simulink model "TCM16QAM_8AMPM"  (Simulink 10.2)
settings: Solver=VariableStepDiscrete  StartTime=0.0  StopTime=1000  RelTol=1e-3  EnableMultiTasking=on
model workspace (MAT data in the model file):
  A = 1
  BER_exit = 0.00293304002933
  BER_th = 0.001
  K = 8
  M = 16
  N = 51
  P_TCM = 10
  P_UNCODED = 10
  T = 1
  ber_TCM = [0.396503893847 0.381864367125 0.373007119222 0.359336876232 0.345566362512 0.327918713861 0.304321668505 0.274140178482 0.213543233397 0.100103613089 0.0215247835823 0.00237307396638 0.000300812192921 0]
  ber_UNCODED = [0.296470352965 0.274672532747 0.252474752525 0.224277572243 0.193513981935 0.163083691631 0.130453621305 0.101523181015 0.0726927307269 0.0482285104823 0.028797120288 0.0161650501617 0.00649935006499 0.00293304002933]
  ber_tcm_bit_coded = [0.462699288078 0.465055650256 0.463952672215 0.456833450316 0.452321267422 0.438884989472 0.415271232327 0.382382432568 0.324476085431 0.173568635315 0.0402085631204 0.00230622681239 0 0]
  ber_tcm_bit_uncoded = [0.2451011378 0.202749683944 0.169325153374 0.140053924506 0.107111756168 0.0906360906361 0.0594071533562 0.0492233646904 0.0336840162422 0.0120903805497 0.00424358158286 0.00165979277739 0.000451218289381 0]
  coded_bit = 3
  coded_bit_conv = [3 4]
  codegen = [1  0  0  0; 0  1  0  0; 0  0  133  171]
  codegen_2 = [133 171]
  constlen = [1 1 7]
  constlen_2 = 7
  generator_c1 = 133
  generator_c2 = 171
  h = 22
  hh = 0
  hws = Simulink.ModelWorkspace
  i = 15
  k = 3
  label_coded = 'TCM16QAM'
  label_uncoded = '8AMPM'
  list : struct (value not decoded)
  m = 4
  mapping_tcm = [-1-1i 3+3i -1+3i 3-1i -3-3i 1+1i -3+1i 1-3i -3+3i 1-1i -3-1i 1+3i -1+1i 3-3i -1-3i 3+1i]
  mapping_uncoded = [-1+3i -3+1i 3+3i 1+1i 3-1i 1-3i -1-1i -3-3i]
  mdl_name = 'TCM16QAM_8AMPM'
  mm = 0
  model = 'model_TCM16QAM_8AMPM'
  n = 10000
  num_states = 64
  register_length = 7
  seed = 208420
  snr = 14
  snr_start = 0
  snr_step = 1
  snr_vec = [0 1 2 3 4 5 6 7 8 9 10 11 12 13 14]
  ss = 0.824
  startTime = [2021 6 12 8 25 12.196]
  stepTime = [2021 6 12 8 25 35.192]
  step_dur = 0.824
  tb = 28
  tout = [9001 9002 9003 9004 9005 9006 9007 9008 9009 9010 9011 9012 ... (1000 elements, 1000x1)]
  trellis.numInputSymbols = 8
  trellis.numOutputSymbols = 16
  trellis.numStates = 64
  trellis.nextStates = [0  32  0  32  0  32  0  32; 0  32  0  32  0  32  0  32; 1  33  1  33  1  33  1  33; 1  33  1  33  1  33  1  33; 2  34  2  34  2  34  2  34; 2  34  2  34  2  34  2  34; 3  35  3  35  3  35  3  35; 3  35  3  35  3  35  3  35; 4  36  4  36  4  36  4  36; 4  36  4  36  4  36  4  36; 5  37  5  37  5  37  5  37; 5  37  5  37  5  37  5  37; 6  38  6  38  6  38  6  38; 6  38  6  38  6  38  6  38; 7  39  7  39  7  39  7  39; 7  39  7  39  7  39  7  39; 8  40  8  40  8  40  8  40; 8  40  8  40  8  40  8  40; 9  41  9  41  9  41  9  41; 9  41  9  41  9  41  9  41; 10  42  10  42  10  42  10  42; 10  42  10  42  10  42  10  42; 11  43  11  43  11  43  11  43; 11  43  11  43  11  43  11  43; 12  44  12  44  12  44  12  44; 12  44  12  44  12  44  12  44; 13  45  13  45  13  45  13  45; 13  45  13  45  13  45  13  45; 14  46  14  46  14  46  14  46; 14  46  14  46  14  46  14  46; 15  47  15  47  15  47  15  47; 15  47  15  47  15  47  15  47; 16  48  16  48  16  48  16  48; 16  48  16  48  16  48  16  48; 17  49  17  49  17  49  17  49; 17  49  17  49  17  49  17  49; 18  50  18  50  18  50  18  50; 18  50  18  50  18  50  18  50; 19  51  19  51  19  51  19  51; 19  51  19  51  19  51  19  51; 20  52  20  52  20  52  20  52; 20  52  20  52  20  52  20  52; 21  53  21  53  21  53  21  53; 21  53  21  53  21  53  21  53; 22  54  22  54  22  54  22  54; 22  54  22  54  22  54  22  54; 23  55  23  55  23  55  23  55; 23  55  23  55  23  55  23  55; 24  56  24  56  24  56  24  56; 24  56  24  56  24  56  24  56; 25  57  25  57  25  57  25  57; 25  57  25  57  25  57  25  57; 26  58  26  58  26  58  26  58; 26  58  26  58  26  58  26  58; 27  59  27  59  27  59  27  59; 27  59  27  59  27  59  27  59; 28  60  28  60  28  60  28  60; 28  60  28  60  28  60  28  60; 29  61  29  61  29  61  29  61; 29  61  29  61  29  61  29  61; 30  62  30  62  30  62  30  62; 30  62  30  62  30  62  30  62; 31  63  31  63  31  63  31  63; 31  63  31  63  31  63  31  63]
  trellis.outputs = [0  3  4  7  10  13  14  17; 3  0  7  4  13  10  17  14; 2  1  6  5  12  11  16  15; 1  2  5  6  11  12  15  16; 0  3  4  7  10  13  14  17; 3  0  7  4  13  10  17  14; 2  1  6  5  12  11  16  15; 1  2  5  6  11  12  15  16; 3  0  7  4  13  10  17  14; 0  3  4  7  10  13  14  17; 1  2  5  6  11  12  15  16; 2  1  6  5  12  11  16  15; 3  0  7  4  13  10  17  14; 0  3  4  7  10  13  14  17; 1  2  5  6  11  12  15  16; 2  1  6  5  12  11  16  15; 3  0  7  4  13  10  17  14; 0  3  4  7  10  13  14  17; 1  2  5  6  11  12  15  16; 2  1  6  5  12  11  16  15; 3  0  7  4  13  10  17  14; 0  3  4  7  10  13  14  17; 1  2  5  6  11  12  15  16; 2  1  6  5  12  11  16  15; 0  3  4  7  10  13  14  17; 3  0  7  4  13  10  17  14; 2  1  6  5  12  11  16  15; 1  2  5  6  11  12  15  16; 0  3  4  7  10  13  14  17; 3  0  7  4  13  10  17  14; 2  1  6  5  12  11  16  15; 1  2  5  6  11  12  15  16; 1  2  5  6  11  12  15  16; 2  1  6  5  12  11  16  15; 3  0  7  4  13  10  17  14; 0  3  4  7  10  13  14  17; 1  2  5  6  11  12  15  16; 2  1  6  5  12  11  16  15; 3  0  7  4  13  10  17  14; 0  3  4  7  10  13  14  17; 2  1  6  5  12  11  16  15; 1  2  5  6  11  12  15  16; 0  3  4  7  10  13  14  17; 3  0  7  4  13  10  17  14; 2  1  6  5  12  11  16  15; 1  2  5  6  11  12  15  16; 0  3  4  7  10  13  14  17; 3  0  7  4  13  10  17  14; 2  1  6  5  12  11  16  15; 1  2  5  6  11  12  15  16; 0  3  4  7  10  13  14  17; 3  0  7  4  13  10  17  14; 2  1  6  5  12  11  16  15; 1  2  5  6  11  12  15  16; 0  3  4  7  10  13  14  17; 3  0  7  4  13  10  17  14; 1  2  5  6  11  12  15  16; 2  1  6  5  12  11  16  15; 3  0  7  4  13  10  17  14; 0  3  4  7  10  13  14  17; 1  2  5  6  11  12  15  16; 2  1  6  5  12  11  16  15; 3  0  7  4  13  10  17  14; 0  3  4  7  10  13  14  17]
  trellis_2.numInputSymbols = 2
  trellis_2.numOutputSymbols = 4
  trellis_2.numStates = 64
  trellis_2.nextStates = [0  32; 0  32; 1  33; 1  33; 2  34; 2  34; 3  35; 3  35; 4  36; 4  36; 5  37; 5  37; 6  38; 6  38; 7  39; 7  39; 8  40; 8  40; 9  41; 9  41; 10  42; 10  42; 11  43; 11  43; 12  44; 12  44; 13  45; 13  45; 14  46; 14  46; 15  47; 15  47; 16  48; 16  48; 17  49; 17  49; 18  50; 18  50; 19  51; 19  51; 20  52; 20  52; 21  53; 21  53; 22  54; 22  54; 23  55; 23  55; 24  56; 24  56; 25  57; 25  57; 26  58; 26  58; 27  59; 27  59; 28  60; 28  60; 29  61; 29  61; 30  62; 30  62; 31  63; 31  63]
  trellis_2.outputs = [0  3; 3  0; 2  1; 1  2; 0  3; 3  0; 2  1; 1  2; 3  0; 0  3; 1  2; 2  1; 3  0; 0  3; 1  2; 2  1; 3  0; 0  3; 1  2; 2  1; 3  0; 0  3; 1  2; 2  1; 0  3; 3  0; 2  1; 1  2; 0  3; 3  0; 2  1; 1  2; 1  2; 2  1; 3  0; 0  3; 1  2; 2  1; 3  0; 0  3; 2  1; 1  2; 0  3; 3  0; 2  1; 1  2; 0  3; 3  0; 2  1; 1  2; 0  3; 3  0; 2  1; 1  2; 0  3; 3  0; 1  2; 2  1; 3  0; 0  3; 1  2; 2  1; 3  0; 0  3]
  uncoded_bit = [1 2]
undefined symbols (not defined in the file): Mnum
libraries: commsink2 x4, commutil2 x4, dspindex x4, commdigbbndam3 x3, commchan3 x2, commcnvcod2 x2, commdigbbndtcm2 x1, commrandsrc2 x1
settings Model: Creator=Diego  LastModifiedBy=diego
settings DataIOCC: LimitDataPoints=on
settings OptimizationCC: ExpressionDepthLimit=2147483647
settings DebuggingCC: SolverPrmCheckMsg=warning  StateNameClashWarn=warning
settings GRTTargetCC: CombineOutputUpdateFcns=on  GRTInterface=off

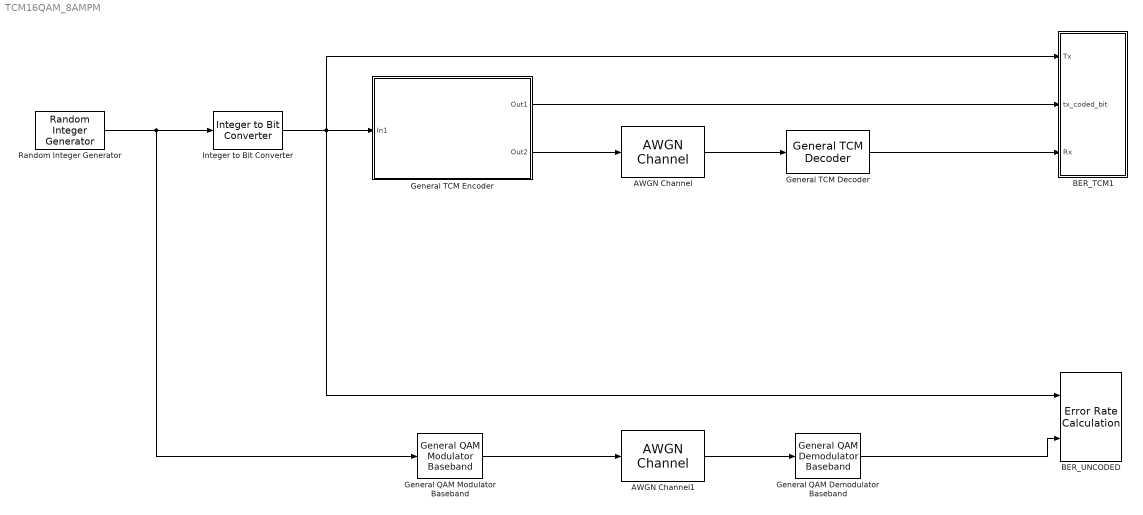
== system TCM16QAM_8AMPM ==
  AWGN Channel : commchan3/AWGN Channel  InputProcessing=Columns as channels (frame based)  seed=seed  noiseMode="Signal to noise ratio  (Es/No)"  EbNodB=Eb_No  EsNodB=snr  SNRdB=snr  bitsPerSym=k  Ps=P_TCM  Tsym=T  variance=1
  AWGN Channel1 : commchan3/AWGN Channel  InputProcessing=Columns as channels (frame based)  seed=seed  noiseMode="Signal to noise ratio  (Es/No)"  EbNodB=Eb_No  EsNodB=snr  SNRdB=snr  bitsPerSym=k  Ps=P_UNCODED  Tsym=1  variance=1
  BER_TCM1 : Subsystem
  BER_UNCODED : commsink2/Error Rate Calculation  N=0  st_delay=0  cp_mode=Entire frame  subframe=[]  PMode=Workspace  WsName=ErrorVec_UNCODED  RsMode2=off  stop=off  numErr=100  maxBits=1e6
  General TCM Decoder : commdigbbndtcm2/General TCM Decoder  trellis=trellis  constpts=mapping_tcm  tbdepth=tb  opmode=Continuous  reset=off  outDtype=double
      settings: SourceProductBaseCode=CM
  General TCM Encoder : Subsystem  AncestorBlock=commdigbbndtcm2/General TCM Encoder  mask(General TCM Encoder){trellis=trellis, opMode=Continuous, constpts=mapping_tcm, outDtype=double}
      mask prompts: trellis "Trellis structure:"; opMode "Operation mode:"; constpts "Signal constellation:"; outDtype "Output data type"
      mask help:
      | Convolutionally encode binary data and perform signal mapping using the Signal constellation parameter, which expects complex constellation points in the set-partitioned order.
      |
      | The Trellis structure parameter must be a valid MATLAB trellis structure. To check if a structure is a valid trellis structure, use the istrellis function in MATLAB.
      mask init:
      | [constpts, Mnum, err, inPortLbl, rstPortLbl] = commblkgentcmenc(gcb, 'init', trellis, constpts);
      | if ~isempty(err.msg)
      | 	error(err.mmi,err.msg);
      | end
      mask Help: helpview(commbhelp)
      mask TypeOptions opMode: Continuous | Truncated (reset every frame) | Terminate trellis by appending bits | Reset on nonzero input via port
      mask TypeOptions outDtype: double | single
      mask Callback outDtype: commblkgentcmenc(gcb, 'cbDtype');
      mask Display:
      | disp('General\nTCM');
      | text(inPortLbl.x, inPortLbl.y, inPortLbl.str);
      | text(rstPortLbl.x, rstPortLbl.y, rstPortLbl.str);
  General QAM Demodulator Baseband : commdigbbndam3/General QAM Demodulator Baseband  SigCon=mapping_uncoded  OutType=Bit  DecType=Hard decision  VarSource=Dialog  Variance=1  outDtypeBit=Inherit via internal rule  outDtype=Inherit via internal rule  roundingMode=Floor  overflowMode=Wrap  OvFlMode=off  OvFlModeLastStrValue=off  sigConstWordLen=16  sigConstDataTypeStr=Inherit: Same word length as input  sigConstLastDataTypeStr=Inherit: Same word length as input  accum1WordLen=32  accum1FracLen=30  prodInWordLen=32  prodInFracLen=30  prodInDataTypeStr=Inherit: Same as accumulator 1  prodInLastDataTypeStr=Inherit: Same as accumulator 1  prodOutWordLen=32  prodOutFracLen=30  accum2WordLen=32  accum2FracLen=30  accum3WordLen=32  accum3FracLen=30  nsiWordLen=32  nsiFracLen=30  nsiDataTypeStr=Inherit: Same as accumulator 3  nsiLastDataTypeStr=Inherit: Same as accumulator 3  invn0WordLen=16  invn0FracLen=8  invn0DataTypeStr=Inherit: Same word length as input  invn0LastDataTypeStr=Inherit: Same word length as input  outputWordLen=32  outputFracLen=30
      settings: SourceProductBaseCode=CM
  General QAM Modulator Baseband : commdigbbndam3/General QAM Modulator Baseband  SigCon=mapping_uncoded  outDtype=double  outWordLen=16  outUDDataType=sfix(16)  outFracLenMode=Best precision  outFracLen=15  outDataTypeStr=double  outLastDataTypeStr=double
      settings: SourceProductBaseCode=CM
  Integer to Bit Converter : commutil2/Integer to Bit Converter  nbits=k  signedInputValues=Unsigned  bitOrder=MSB first  outDtype=Inherit via internal rule
  Random Integer Generator : commrandsrc2/Random Integer Generator  mul=K  seed=seed  Ts=1  frameBased=off  sampPerFrame=frame  orient=off  outDataType=double
      settings: SourceProductBaseCode=CM
  wires:
  Random Integer Generator/1 -> Integer to Bit Converter/1, General QAM Modulator Baseband/1
  Integer to Bit Converter/1 -> BER_UNCODED/1, General TCM Encoder/1(In1), BER_TCM1/1(Tx)
  AWGN Channel/1 -> General TCM Decoder/1
  General QAM Modulator Baseband/1 -> AWGN Channel1/1
  AWGN Channel1/1 -> General QAM Demodulator Baseband/1
  General QAM Demodulator Baseband/1 -> BER_UNCODED/2
  General TCM Encoder/2(Out2) -> AWGN Channel/1
  General TCM Encoder/1(Out1) -> BER_TCM1/2(tx_coded_bit)
  General TCM Decoder/1 -> BER_TCM1/3(Rx)

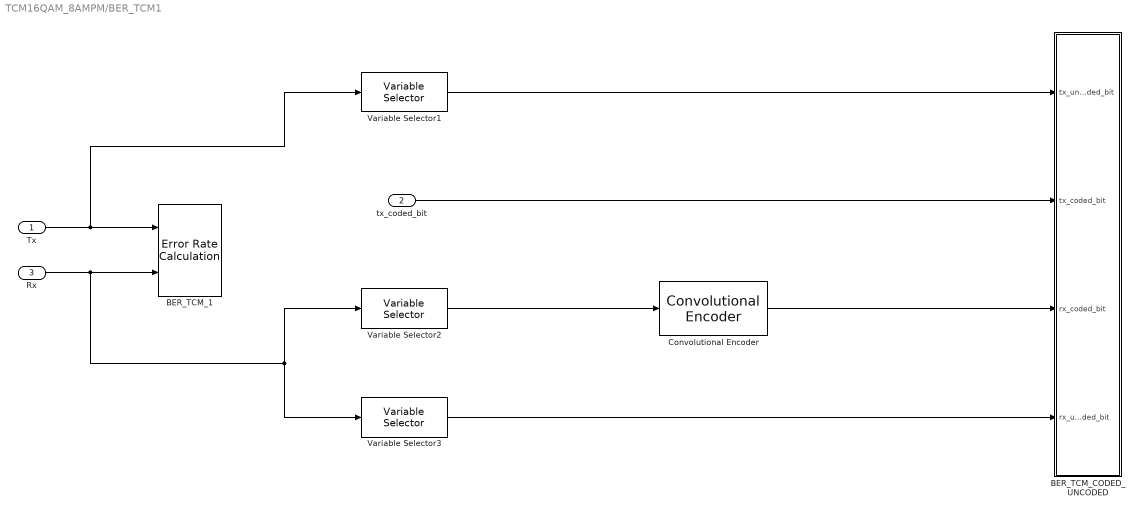
== system TCM16QAM_8AMPM/BER_TCM1 ==
  Tx : Inport
  tx_coded_bit : Inport  Port=2
  Rx : Inport  Port=3
  BER_TCM_1 : commsink2/Error Rate Calculation  N=tb*k  st_delay=0  cp_mode=Entire frame  subframe=[]  PMode=Workspace  WsName=ErrorVec_TCM_1  RsMode2=off  stop=off  numErr=100  maxBits=1e6
  BER_TCM_CODED_UNCODED : Subsystem
  Convolutional Encoder : commcnvcod2/Convolutional Encoder  trellis=trellis_2  opMode=Continuous  DelayedResetAction=off  hasIniStPort=off  hasFinStPort=off  usePuncVector=off  punctureVector=[1; 1; 0; 1; 0; 1]  reset=Unused parameter value
      settings: SourceProductBaseCode=CM
  Variable Selector1 : dspindex/Variable Selector  NumInputs=1  rowsOrCols=Rows  IdxMode=Fixed  Elements=uncoded_bit  ZerOneIdxMode=One-based  errmode=Clip Index  FillMode=on  FillValues=0
  Variable Selector2 : dspindex/Variable Selector  NumInputs=1  rowsOrCols=Rows  IdxMode=Fixed  Elements=coded_bit  ZerOneIdxMode=One-based  errmode=Clip Index  FillMode=on  FillValues=0
  Variable Selector3 : dspindex/Variable Selector  NumInputs=1  rowsOrCols=Rows  IdxMode=Fixed  Elements=uncoded_bit  ZerOneIdxMode=One-based  errmode=Clip Index  FillMode=on  FillValues=0
  wires:
  Tx/1 -> BER_TCM_1/1, Variable Selector1/1
  Rx/1 -> BER_TCM_1/2, Variable Selector2/1, Variable Selector3/1
  Variable Selector1/1 -> BER_TCM_CODED_UNCODED/1(tx_uncoded_bit)
  Variable Selector2/1 -> Convolutional Encoder/1
  Variable Selector3/1 -> BER_TCM_CODED_UNCODED/4(rx_uncoded_bit)
  tx_coded_bit/1 -> BER_TCM_CODED_UNCODED/2(tx_coded_bit)
  Convolutional Encoder/1 -> BER_TCM_CODED_UNCODED/3(rx_coded_bit)

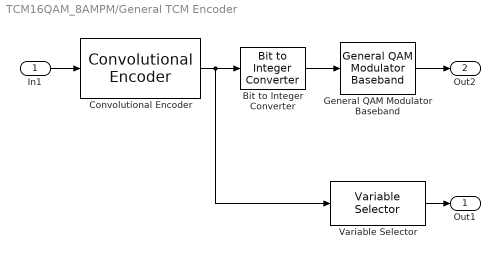
== system TCM16QAM_8AMPM/General TCM Encoder ==
  In1 : Inport
  Bit to Integer Converter : commutil2/Bit to Integer Converter  nbits=log2(Mnum)  bitOrder=MSB first  signedOutputValues=Unsigned  outDtype=uint32  outDtypeSigned=Inherit via internal rule
  Convolutional Encoder : commcnvcod2/Convolutional Encoder  trellis=trellis  opMode=Continuous  DelayedResetAction=off  hasIniStPort=off  hasFinStPort=off  usePuncVector=off  punctureVector=[1; 1; 0; 1; 0; 1]  reset=Unused parameter value
      settings: SourceProductBaseCode=CM
  General QAM Modulator Baseband : commdigbbndam3/General QAM Modulator Baseband  SigCon=constpts  outDtype=double  outWordLen=16  outUDDataType=sfix(16)  outFracLenMode=Best precision  outFracLen=15  outDataTypeStr=double  outLastDataTypeStr=double
      settings: SourceProductBaseCode=CM
  Variable Selector : dspindex/Variable Selector  NumInputs=1  rowsOrCols=Rows  IdxMode=Fixed  Elements=coded_bit_conv  ZerOneIdxMode=One-based  errmode=Clip Index  FillMode=on  FillValues=0
  Out1 : Outport
  Out2 : Outport  Port=2
  wires:
  Bit to Integer Converter/1 -> General QAM Modulator Baseband/1
  In1/1 -> Convolutional Encoder/1
  Convolutional Encoder/1 -> Bit to Integer Converter/1, Variable Selector/1
  General QAM Modulator Baseband/1 -> Out2/1
  Variable Selector/1 -> Out1/1

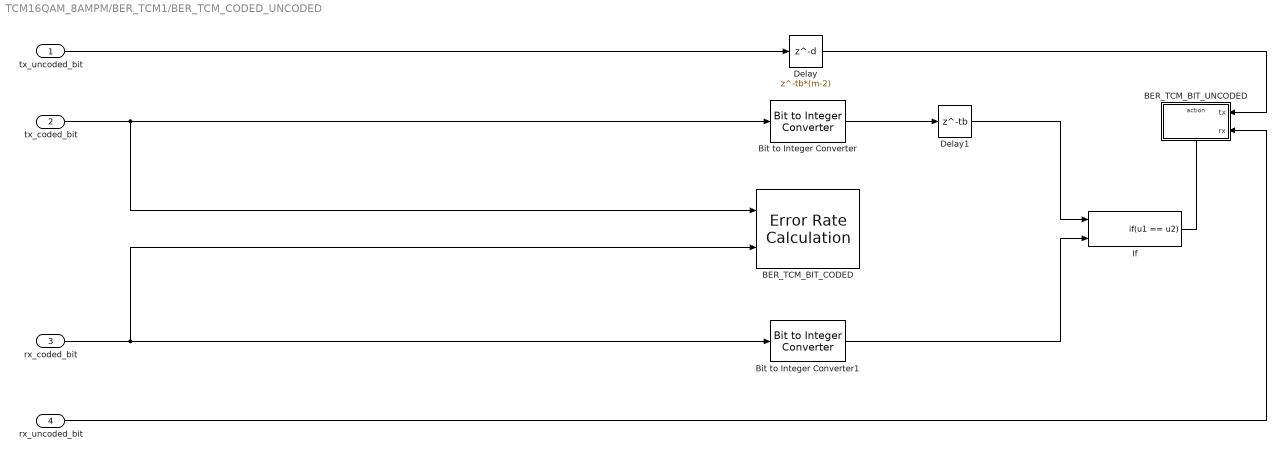
== system TCM16QAM_8AMPM/BER_TCM1/BER_TCM_CODED_UNCODED ==
  tx_uncoded_bit : Inport
  tx_coded_bit : Inport  Port=2
  rx_coded_bit : Inport  Port=3
  rx_uncoded_bit : Inport  Port=4
  BER_TCM_BIT_CODED : commsink2/Error Rate Calculation  N=tb*2  st_delay=0  cp_mode=Entire frame  subframe=[]  PMode=Workspace  WsName=ErrorVec_TCM_COD_1  RsMode2=off  stop=off  numErr=100  maxBits=1e6
  BER_TCM_BIT_UNCODED : Subsystem  TreatAsAtomicUnit=on
  Bit to Integer Converter : commutil2/Bit to Integer Converter  nbits=2  bitOrder=MSB first  signedOutputValues=Unsigned  outDtype=Inherit via internal rule  outDtypeSigned=Inherit via internal rule
  Bit to Integer Converter1 : commutil2/Bit to Integer Converter  nbits=2  bitOrder=MSB first  signedOutputValues=Unsigned  outDtype=Inherit via internal rule  outDtypeSigned=Inherit via internal rule
  Delay : Delay  DelayLength=tb*(m-2)  InputProcessing=Columns as channels (frame based)
  Delay1 : Delay  DelayLength=tb  InputProcessing=Columns as channels (frame based)
  If : If  NumInputs=2  IfExpression=u1 == u2  ShowElse=off
  wires:
  tx_uncoded_bit/1 -> Delay/1
  tx_coded_bit/1 -> BER_TCM_BIT_CODED/1, Bit to Integer Converter/1
  rx_coded_bit/1 -> BER_TCM_BIT_CODED/2, Bit to Integer Converter1/1
  Delay/1 -> BER_TCM_BIT_UNCODED/1(tx)
  rx_uncoded_bit/1 -> BER_TCM_BIT_UNCODED/2(rx)
  If/1 -> BER_TCM_BIT_UNCODED/Action
  Bit to Integer Converter/1 -> Delay1/1
  Bit to Integer Converter1/1 -> If/2
  Delay1/1 -> If/1

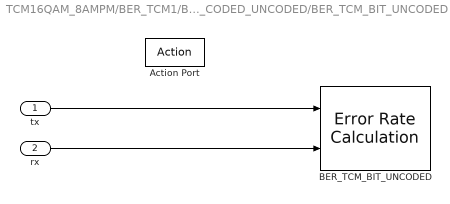
== system TCM16QAM_8AMPM/BER_TCM1/BER_TCM_CODED_UNCODED/BER_TCM_BIT_UNCODED ==
  tx : Inport
  rx : Inport  Port=2
  Action Port : ActionPort  ActionPortLabel=if(u1 == u2)
  BER_TCM_BIT_UNCODED : commsink2/Error Rate Calculation  N=0  st_delay=tb*(m-2)  cp_mode=Entire frame  subframe=[]  PMode=Workspace  WsName=ErrorVec_TCM_bit_uncoded  RsMode2=off  stop=off  numErr=100  maxBits=1e6
  wires:
  tx/1 -> BER_TCM_BIT_UNCODED/1
  rx/1 -> BER_TCM_BIT_UNCODED/2
